simulink subsystem "Controller"  (R2020a)
settings: Solver=VariableStepAuto  StartTime=0.0  StopTime=10.0  RelTol=1e-3
values from neighbouring files (symbols this model uses):
  Eqlut = zeros(slotsAngle, slotsSpeed, 2)    [LUTScript.m]    (also in Lutscript.m = zeros(10,13,2); generateLUTs.m)
  Klut = zeros(slotsAngle, slotsSpeed, 2)    [LUTScript.m]    (also in Lutscript.m = zeros(10,13,2); generateLUTs.m)
  maxAngle = 30    [SimRoutine.m]    (also in SimRoutine2.m; generateLUTs.m)
  maxSpeed = 200    [SimRoutine.m]    (also in SimRoutine2.m; generateLUTs.m)
  resAngle = 3    [SimRoutine.m]    (also in SimRoutine2.m; generateLUTs.m)
  resSpeed = 10    [SimRoutine.m]    (also in SimRoutine2.m; generateLUTs.m)
  thrAngle = ((resAngle*2)/100) * 10    (= 0.6)    [SimRoutine2.m]
  thrSpeed = ((resSpeed*2)/100) * 10    (= 2)    [SimRoutine2.m]
  VEH = getVariable(get_param(bdroot('CRReferenceApplication'), 'modelworkspace'),'VEH')    [SimRoutine.m]    (also in SimRoutine2.m; SimRoutuine.m)
settings Model: Creator=Fil  LastModifiedBy=filip

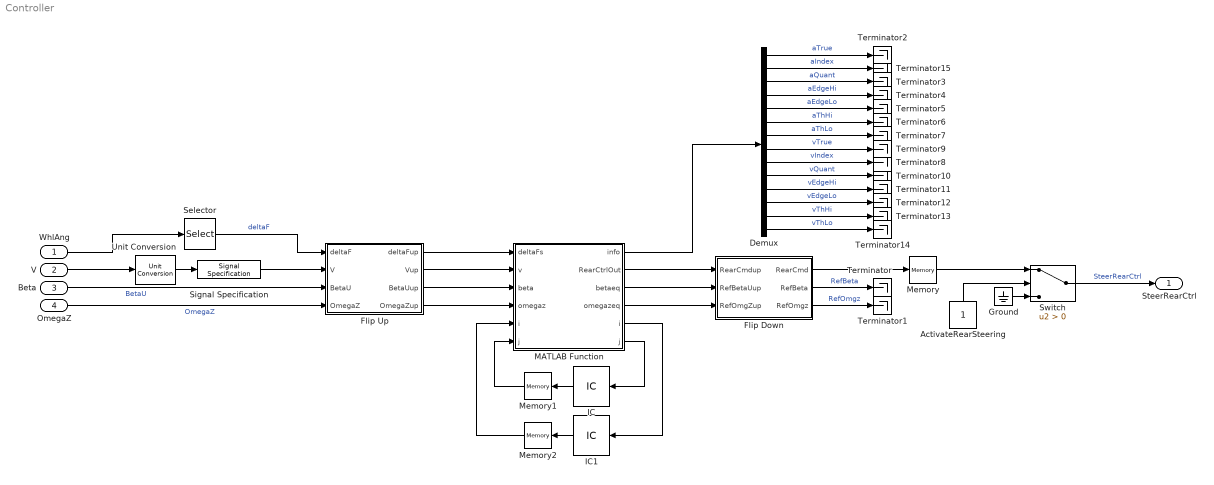
== system Controller ==
  WhlAng : Inport
  V : Inport  Port=2
  Beta : Inport  Port=3
  OmegaZ : Inport  Port=4
  ActivateRearSteering : Constant
  Demux : Demux  Outputs=14
  Flip Down : Subsystem
  Flip Up : Subsystem
  Ground : Ground
  IC : InitialCondition  Value=0
  IC1 : InitialCondition  Value=0
  MATLAB Function : MATLAB Function  TreatAsAtomicUnit=on
      settings: MinAlgLoopOccurrences=on
  Memory : Memory
  Memory1 : Memory
  Memory2 : Memory
  Selector : Selector  InputPortWidth=4  IndexOptions=Index vector (dialog)  Indices=[1 2]  OutputSizes=1
  Signal Specification : SignalSpecification  Unit=km/h
  Switch : Switch  Criteria=u2 > Threshold
  Terminator{,1..15} (16 alike) : Terminator
  Unit Conversion : UnitConversion
  SteerRearCtrl : Outport
  wires:
  WhlAng/1 -> Selector/1
  Memory/1 -> Switch/1
  ActivateRearSteering/1 -> Switch/2
  Switch/1 -> SteerRearCtrl/1  "SteerRearCtrl"
  Ground/1 -> Switch/3
  Selector/1 -> Flip Up/1(deltaF)  "deltaF"
  V/1 -> Unit Conversion/1
  Beta/1 -> Flip Up/3(BetaU)  "BetaU"
  OmegaZ/1 -> Flip Up/4(OmegaZ)  "OmegaZ"
  Flip Up/1(deltaFup) -> MATLAB Function/1(deltaFs)
  Flip Up/2(Vup) -> MATLAB Function/2(v)
  Flip Up/3(BetaUup) -> MATLAB Function/3(beta)
  Flip Up/4(OmegaZup) -> MATLAB Function/4(omegaz)
  MATLAB Function/2(RearCtrlOut) -> Flip Down/1(RearCmdup)
  MATLAB Function/3(betaeq) -> Flip Down/2(RefBetaUup)
  MATLAB Function/4(omegazeq) -> Flip Down/3(RefOmgZup)
  Flip Down/1(RearCmd) -> Memory/1
  Flip Down/2(RefBeta) -> Terminator/1  "RefBeta"
  Flip Down/3(RefOmgz) -> Terminator1/1  "RefOmgz"
  Memory1/1 -> MATLAB Function/6("j ")
  Memory2/1 -> MATLAB Function/5("i ")
  IC1/1 -> Memory2/1
  IC/1 -> Memory1/1
  MATLAB Function/6(j) -> IC/1
  MATLAB Function/5(i) -> IC1/1
  Unit Conversion/1 -> Signal Specification/1
  Signal Specification/1 -> Flip Up/2(V)
  MATLAB Function/1(info) -> Demux/1
  Demux/1 -> Terminator2/1  "aTrue"
  Demux/3 -> Terminator3/1  "aQuant"
  Demux/4 -> Terminator4/1  "aEdgeHi"
  Demux/5 -> Terminator5/1  "aEdgeLo"
  Demux/6 -> Terminator6/1  "aThHi"
  Demux/7 -> Terminator7/1  "aThLo"
  Demux/8 -> Terminator9/1  "vTrue"
  Demux/10 -> Terminator10/1  "vQuant"
  Demux/11 -> Terminator11/1  "vEdgeHi"
  Demux/12 -> Terminator12/1  "vEdgeLo"
  Demux/13 -> Terminator13/1  "vThHi"
  Demux/14 -> Terminator14/1  "vThLo"
  Demux/9 -> Terminator8/1  "vIndex"
  Demux/2 -> Terminator15/1  "aIndex"

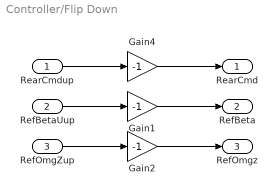
== system Controller/Flip Down ==
  RearCmdup : Inport
  RefBetaUup : Inport  Port=2
  RefOmgZup : Inport  Port=3
  Gain1 : Gain  Gain=-1
  Gain2 : Gain  Gain=-1
  Gain4 : Gain  Gain=-1
  RearCmd : Outport
  RefBeta : Outport  Port=2
  RefOmgz : Outport  Port=3
  wires:
  Gain4/1 -> RearCmd/1
  Gain1/1 -> RefBeta/1
  RefBetaUup/1 -> Gain1/1
  RefOmgZup/1 -> Gain2/1
  RearCmdup/1 -> Gain4/1
  Gain2/1 -> RefOmgz/1

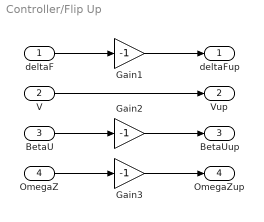
== system Controller/Flip Up ==
  deltaF : Inport
  V : Inport  Port=2
  BetaU : Inport  Port=3
  OmegaZ : Inport  Port=4
  Gain1 : Gain  Gain=-1
  Gain2 : Gain  Gain=-1
  Gain3 : Gain  Gain=-1
  deltaFup : Outport
  Vup : Outport  Port=2
  BetaUup : Outport  Port=3
  OmegaZup : Outport  Port=4
  wires:
  deltaF/1 -> Gain1/1
  Gain1/1 -> deltaFup/1
  V/1 -> Vup/1
  Gain3/1 -> OmegaZup/1
  OmegaZ/1 -> Gain3/1
  BetaU/1 -> Gain2/1
  Gain2/1 -> BetaUup/1

== matlab function Controller/MATLAB Function ==
  data: info output; deltaFs input; RearCtrlOut output; v input; beta input; omegaz input; i input; j input; Klut parameter; Eqlut parameter; resAngle parameter; resSpeed parameter; betaeq output; omegazeq output; maxSpeed parameter; maxAngle parameter; thrAngle parameter; thrSpeed parameter; i output; j output; VEH parameter
function [info, RearCtrlOut,betaeq,omegazeq, i, j] = optRear(deltaFs,v,beta,omegaz, i, j, Klut, Eqlut, resAngle, resSpeed, maxSpeed, maxAngle, thrAngle, thrSpeed, VEH)

    K   = zeros(2);
    Ref = zeros(2);
    
    
    % Select LUT indexes (w/ Schmitt Trigger):
    % If well beyond the previous sub-range, with added guard threshold...
        % ...pick the LUT index centered around the new sub-range.

    deltaF = mean(deltaFs);
    aTrue = rad2deg(abs(deltaF));
    if aTrue > maxAngle
        aTrue = maxAngle;
    end
    aIndex = floor( (aTrue + resAngle/2) / resAngle );
    aQuant = aIndex * resAngle;
    aEdgeHi = i*resAngle + resAngle/2;
    aEdgeLo = i*resAngle - resAngle/2;
    aThHi = (aEdgeHi + thrAngle);
    aThLo = (aEdgeLo - thrAngle);
    
    if aTrue < aThLo | aTrue > aThHi
        i = aIndex;
    end
    
    
    vTrue = abs(v);
    if vTrue > maxSpeed
        vTrue = maxSpeed;
    end
    vIndex = floor( (vTrue + resSpeed/2) / resSpeed );
    vQuant = vIndex * resSpeed;
    vEdgeHi = j*resSpeed + resSpeed/2;
    vEdgeLo = j*resSpeed - resSpeed/2;
    vThHi = (vEdgeHi + thrSpeed);
    vThLo = (vEdgeLo - thrSpeed);
    
    if vTrue < vThLo | vTrue > vThHi
        j = vIndex;
    end
    
    info = [aTrue, aIndex, aQuant, aEdgeHi, aEdgeLo, aThHi, aThLo, vTrue, vIndex, vQuant, vEdgeHi, vEdgeLo, vThHi, vThLo];
    
    
    % Infer equilibrium point
    CfRaw = 15000;
    CrRaw = 35000;
    
    muL0 = 0;
    for mu = 1:4
        muL0 = muL0 + Partial_mu_long(mu,0);
    end
    muL0 = muL0/4;
    muL0 = 0.8;
    
    rxf = VEH.FrontAxlePositionfromCG;      % Front Wheels X Axis Offset (Length)
    rxr = -(VEH.RearAxlePositionfromCG);    % Rear Wheels X Axis Offset (Length)
    Iz = VEH.YawMomentInertia;
    m = VEH.Mass;
    ryf = VEH.TrackWidth/2;
    g = 9.81;
    
    if (v<1)    % Divide-by-Zero safeguard
        v = 1;
    end
    v = v/3.6;  % [km/h] --> [m/s]
    
    lf = sqrt(rxf^2+ryf^2);
    lr = sqrt(rxr^2+ryf^2);
    Cf = muL0*CfRaw;
    Cr = muL0*CrRaw;
    A11 = -(Cf+Cr);
    A12 = -m*v-(Cf*rxf+Cr*rxr)/(v);
    A21 = -(Cf*rxf+Cr*rxr);
    A22 = -(Cf*lf^2+Cr*lr^2)/(v);
    A = [1/(m*v) 0;0 1/Iz]*[A11 A12; A21 A22];
    B2 = [1/(m*v) 0;0 1/Iz]*[Cf; Cf*rxf];
    xeq = (inv(A))*[-B2*(deltaF)];
    if abs(xeq(2)) > 0.85*1.3*g/v
        xeq(2) = 0.85*1.3*g/v * sign(xeq(2));
    end
    if abs(xeq(1)) > atan(0.02*1.3*g)
        xeq(1) = atan(0.02*1.3*g) * sign(xeq(1));
    end
    Ref = xeq;
    %omegaZack = (v/(rxf-rxr))*tan(deltaF);
    %xeq(2,1) = omegaZack;

    % Extract from LUTs
    K   =  Klut(i+1, j+1, :);
    %Ref = Eqlut(i+1, j+1, :);
    
    % Equilibrium references from LUT, matching sign to turn direction
    betaeq   = 0;     %sign(deltaF);
    omegazeq = Ref(2);%sign(deltaF);
    
    % Control signal output u = -Kx
    RearCtrlOut = -((K(1)*(beta-betaeq)) + (K(2)*(omegaz-omegazeq)));
end
